simulink model "SimpleBatterySimulation"  (R2020a)
settings: Solver=VariableStepAuto  StartTime=0.0  StopTime=3600  RelTol=1e-3
values from neighbouring files (symbols this model uses):
  Cn = 2.3*3600    (= 8280)    [SimpleBatteryScript.m]
  I = -2.3    [SimpleBatteryScript.m]
  OCV = Data(:,2)    [SimpleBatteryScript.m]
  R_Charge = Data(:,3)    [SimpleBatteryScript.m]
  R_Discharge = Data(:,4)    [SimpleBatteryScript.m]
  SOC = Data(:,1)    [SimpleBatteryScript.m]
settings Model: Creator=diogo  LastModifiedBy=diogo

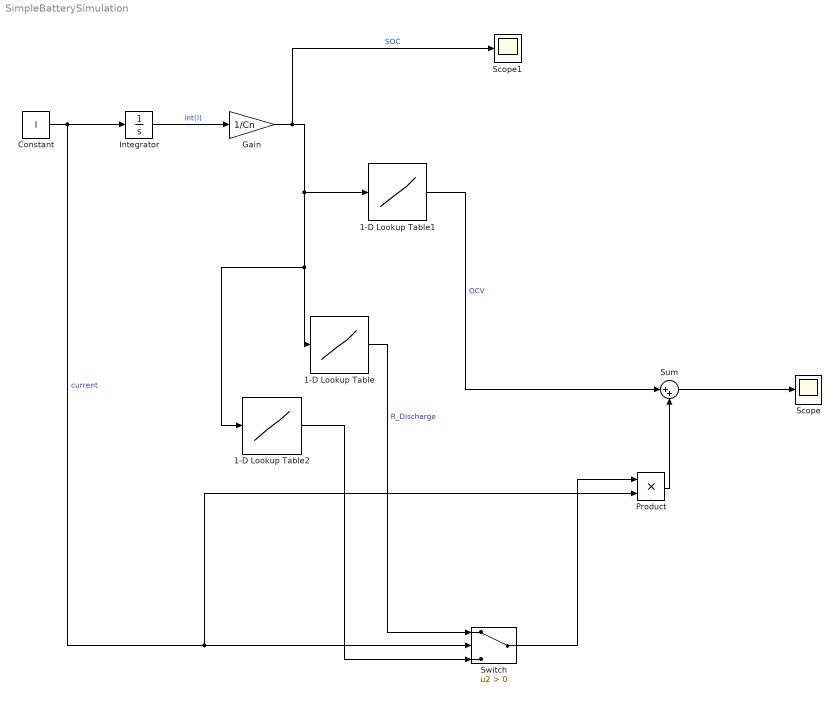
== system SimpleBatterySimulation ==
  1-D Lookup Table : Lookup_n-D  NumberOfTableDimensions=1  BreakpointsForDimension1=SOC  Table=R_Discharge  InternalRulePriority=Speed  RndMeth=Simplest  InputSameDT=on
  1-D Lookup Table1 : Lookup_n-D  NumberOfTableDimensions=1  BreakpointsForDimension1=SOC  Table=OCV  InternalRulePriority=Speed  RndMeth=Simplest  InputSameDT=on
  1-D Lookup Table2 : Lookup_n-D  NumberOfTableDimensions=1  BreakpointsForDimension1=SOC  Table=R_Charge  InternalRulePriority=Speed  RndMeth=Simplest  InputSameDT=on
  Constant : Constant  Value=I
  Gain : Gain  Gain=1/Cn
  Integrator : Integrator
  Product : Product
  Scope : Scope
  Scope1 : Scope
  Sum : Sum  Inputs=|++
  Switch : Switch  Criteria=u2 > Threshold
  wires:
  Constant/1 -> Product/2, Switch/2, Integrator/1  "current"
  Integrator/1 -> Gain/1  "int(I)"
  Gain/1 -> Scope1/1, 1-D Lookup Table1/1, 1-D Lookup Table2/1, 1-D Lookup Table/1  "SOC"
  Product/1 -> Sum/2
  Sum/1 -> Scope/1
  1-D Lookup Table1/1 -> Sum/1  "OCV"
  Switch/1 -> Product/1
  1-D Lookup Table/1 -> Switch/1  "R_Discharge"
  1-D Lookup Table2/1 -> Switch/3
